simulink model "RT_ueb3_2d"  (R2013a)
settings: Solver=ode45  StartTime=0.0  StopTime=10.0  RelTol=1e-3
values from neighbouring files (symbols this model uses):
  k = 2    [rt_uebung2_post.m]
undefined symbols (not defined in the file or in its folder): n0, n1
settings Model: BufferReuse=off  Creator=mainster  LastModifiedBy=mainster
settings OptimizationCC: InlineParams=on  BufferReuse=off
settings DebuggingCC: InitInArrayFormatMsg=none

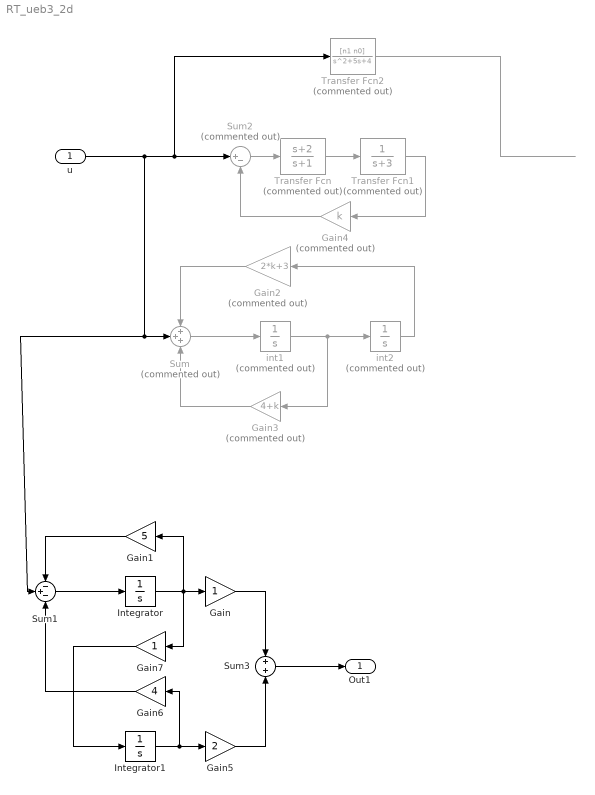
== system RT_ueb3_2d ==
  u : Inport
  Gain : Gain
  Gain1 : Gain  Gain=5
  Gain2 : Gain  Commented=on  Gain=2*k+3
  Gain3 : Gain  Commented=on  Gain=4+k
  Gain4 : Gain  Commented=on  Gain=k
  Gain5 : Gain  Gain=2
  Gain6 : Gain  Gain=4
  Gain7 : Gain
  Integrator : Integrator
  Integrator1 : Integrator
  Sum : Sum  Commented=on  Inputs=+++
  Sum1 : Sum  Inputs=-+-
  Sum2 : Sum  Commented=on  Inputs=|+-
  Sum3 : Sum  Inputs=+|+
  Transfer Fcn : TransferFcn  Commented=on  Numerator=[1 2]  Denominator=[1 1]
  Transfer Fcn1 : TransferFcn  Commented=on  Denominator=[1 3]
  Transfer Fcn2 : TransferFcn  Commented=on  Numerator=[n1 n0]  Denominator=[1 5 4]
  int1 : Integrator  Commented=on  InitialCondition=1
  int2 : Integrator  Commented=on  InitialCondition=1
  Out1 : Outport
  wires:
  Sum/1 -> int1/1
  int1/1 -> Gain3/1, int2/1
  Gain2/1 -> Sum/1
  int2/1 -> Gain2/1
  Gain3/1 -> Sum/3
  Transfer Fcn/1 -> Transfer Fcn1/1
  Sum2/1 -> Transfer Fcn/1
  u/1 -> Sum1/2, Sum/2, Transfer Fcn2/1, Sum2/1
  Gain4/1 -> Sum2/2
  Transfer Fcn1/1 -> Gain4/1
  Transfer Fcn2/1 -> ?
  Sum1/1 -> Integrator/1
  Integrator/1 -> Gain7/1, Gain1/1, Gain/1
  Gain/1 -> Sum3/1
  Gain5/1 -> Sum3/2
  Integrator1/1 -> Gain6/1, Gain5/1
  Gain6/1 -> Sum1/3
  Gain1/1 -> Sum1/1
  Gain7/1 -> Integrator1/1
  Sum3/1 -> Out1/1
